simulink model "ee463_project_simulation vol2"  (R2023b)
settings: Solver=VariableStepAuto  StartTime=0.0  StopTime=0.20  RelTol=1e-3
undefined symbols (not defined in the file or in its folder): Acid, Lead
libraries: spsDiodeLib x8, spsACVoltageSourceLib x3, spsSeriesRLCBranchLib x3, spsVoltageMeasurementLib x3, spsBatteryLib x1, spsCurrentMeasurementLib x1, spsGroundLib x1, spsMeanLib x1, spsMosfetLib x1, sps_lib x1
settings Model: Creator=Emir  LastModifiedBy=Emir

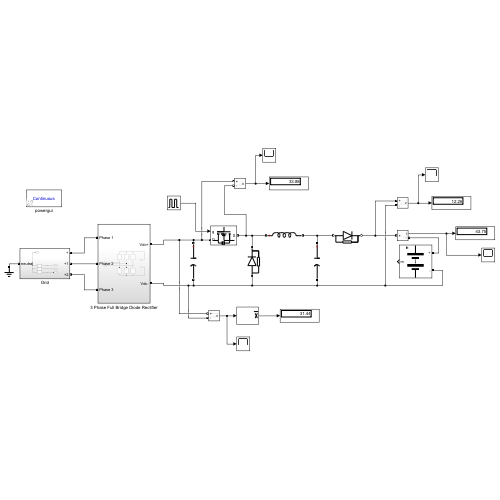
[thumbnail: Simulink's stored preview of the top-level diagram]
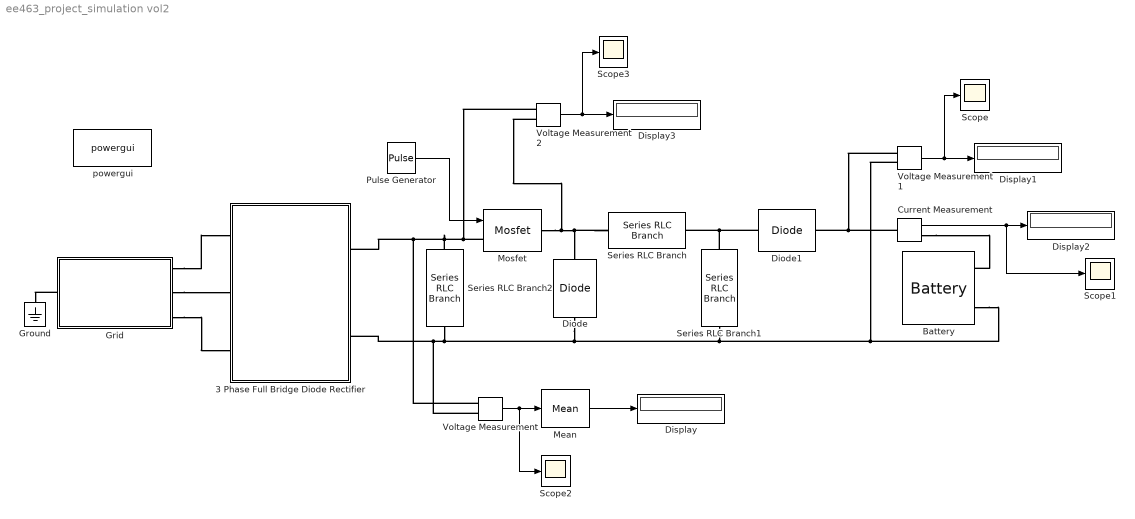
== system ee463_project_simulation vol2 ==
  3 Phase Full Bridge Diode Rectifier : Subsystem
  Battery : spsBatteryLib/Battery  BatType=Lead-Acid  ShowTempParam=off  ThermalPreset=no  ShowAgeParam=off  NomV=12  NomQ=100  SOC=80  Batt_Tr=30  PresetModel=on  MaxQ=104.1667  MinV=9  FullV=13.0658  Dis_rate=20  R=0.0012  Normal_OP=31.0278  expZone="[12.2171     0.333333]"  current=[6.5 13 32.5]  Units=Time  Tci=20  NomT=20  T2=-30  MaxQ2=4.8  FullV2=7.1  Normal_OP2=5.655  expZone2="[6.58           1]"  Rca=0.6  ti=2000  Dp=0  Neq0=0  Tsim=1e6  Ta1=25  Qeol=5.4*0.9  Reol=0.013333*1.2  Char_age=[2.3478, 3]  Dis_age=[2.3478, 10]  N1=1500  N2=10500  N3=1000  N4=1400  Ta2=45  N5=950
  Current Measurement : spsCurrentMeasurementLib/Current Measurement  PhasorSimulation=off  OutputType=Complex  PSBequivalent=0
  Diode : spsDiodeLib/Diode  Ron=0.001  Lon=0  Vf=0.8  IC=0  UseSnubber=0  Rs=500  Cs=250e-9  Measurements=off
  Diode1 : spsDiodeLib/Diode  Ron=0.001  Lon=0  Vf=0.8  IC=0  UseSnubber=0  Rs=500  Cs=250e-9  Measurements=off
  Display{,1..3} (4 alike) : Display
  Grid : Subsystem
  Ground : spsGroundLib/Ground  LConnTagsString=a
  Mean : spsMeanLib/Mean  Freq=60  Vinit=0  Ts=0
  Mosfet : spsMosfetLib/Mosfet  Ron=0.1  Lon=0  Rd=0.01  Vfd=0  IC=0  Rs=1e5  Cs=inf  Measurements=off
  Pulse Generator : DiscretePulseGenerator  PulseType=Time based  Period=1e-5  PulseWidth=50
  Scope{,1..3} (4 alike) : Scope
  Series RLC Branch : spsSeriesRLCBranchLib/Series RLC Branch  LConnTagsString=__new0  RConnTagsString=__new0  BranchType=L  Resistance=1  Inductance=1e-3  SetiL0=off  InitialCurrent=0  Capacitance=1e-6  Setx0=off  InitialVoltage=0  Measurements=None
  Series RLC Branch1 : spsSeriesRLCBranchLib/Series RLC Branch  LConnTagsString=__new0  RConnTagsString=__new0  BranchType=C  Resistance=100  Inductance=1e-3  SetiL0=off  InitialCurrent=0  Capacitance=1000e-6  Setx0=off  InitialVoltage=0  Measurements=None
  Series RLC Branch2 : spsSeriesRLCBranchLib/Series RLC Branch  LConnTagsString=__new0  RConnTagsString=__new0  BranchType=C  Resistance=100  Inductance=1e-3  SetiL0=off  InitialCurrent=0  Capacitance=1000e-6  Setx0=off  InitialVoltage=0  Measurements=None
  Voltage Measurement : spsVoltageMeasurementLib/Voltage Measurement  PhasorSimulation=off  OutputType=Complex  PSBequivalent=0
  Voltage Measurement1 : spsVoltageMeasurementLib/Voltage Measurement  PhasorSimulation=off  OutputType=Complex  PSBequivalent=0
  Voltage Measurement2 : spsVoltageMeasurementLib/Voltage Measurement  PhasorSimulation=off  OutputType=Complex  PSBequivalent=0
  powergui : sps_lib/powergui  Priority=1  SimulationMode=Continuous  SampleTime=50e-6  frequency=60  Iterations=50  frequencyindice=50  Pbase=100e6  ErrMax=1e-4  UnitsV=kV  UnitsW=MW  buscounter=0  FunctionMessages=off  echomessages=off  EnableUseOfTLC=off  CurrentSourceSwitches=off  DisableSnubberDevices=off  DisableRonSwitches=off  DisableVfSwitches=off  DisplayEquations=off  AutomaticDiscreteSolvers=off  SolverType=Tustin/Backward Euler (TBE)  Interpol=off  ExternalGateDelay=off  methode=off  Ts=100  x0status=blocks  SPID=on  SwTol=0  HookPort=off  NonlinearTolerance=1e-4  nMaxIteration=100  ContinueOnMaxIteration=off  RestoreLinks=warning  ResistiveCurrentMeasurement=off  Frange=[0:2:500]  Ylog=off  Xlog=on  ShowGrid=off  save=off  variable=ZData  structure=0  ZoomFFT=off  StartTime=0.0  cycles=1  DisplayStyle=1  fundamental=60  FreqAxis=off  MaxFrequency=1000  frequencyindicesteady=1  RmsSteady=1  display=off
  wires:
  Voltage Measurement/1 -> Scope2/1, Mean/1
  Mean/1 -> Display/1
  Voltage Measurement1/1 -> Scope/1, Display1/1
  Current Measurement/1 -> Scope1/1, Display2/1
  Pulse Generator/1 -> Mosfet/1
  Voltage Measurement2/1 -> Display3/1, Scope3/1
  connections:
  Series RLC Branch2/RConn1 -- Voltage Measurement1/LConn2 -- Battery/LConn2 -- Series RLC Branch1/RConn1 -- Diode/LConn1 -- Voltage Measurement/LConn2 -- 3 Phase Full Bridge Diode Rectifier/RConn2
  Grid/RConn1 -- 3 Phase Full Bridge Diode Rectifier/LConn1
  Grid/RConn2 -- 3 Phase Full Bridge Diode Rectifier/LConn2
  Grid/RConn3 -- 3 Phase Full Bridge Diode Rectifier/LConn3
  Grid/LConn1 -- Ground/LConn1
  Series RLC Branch2/LConn1 -- Voltage Measurement2/LConn1 -- Mosfet/LConn1 -- Voltage Measurement/LConn1 -- 3 Phase Full Bridge Diode Rectifier/RConn1
  Mosfet/RConn1 -- Voltage Measurement2/LConn2 -- Diode/RConn1 -- Series RLC Branch/LConn1
  Series RLC Branch1/LConn1 -- Diode1/LConn1 -- Series RLC Branch/RConn1
  Voltage Measurement1/LConn1 -- Current Measurement/LConn1 -- Diode1/RConn1
  Current Measurement/RConn1 -- Battery/LConn1

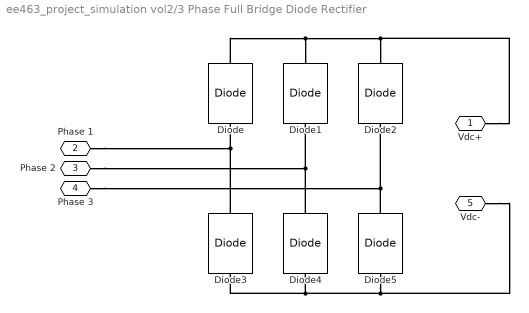
== system ee463_project_simulation vol2/3 Phase Full Bridge Diode Rectifier ==
  Diode{,1..5} (6 alike) : spsDiodeLib/Diode  Ron=0.001  Lon=0  Vf=0.8  IC=0  UseSnubber=0  Rs=500  Cs=250e-9  Measurements=off
  Vdc+ : PMIOPort  Side=Right
  Phase 1 : PMIOPort  Port=2  Side=Left
  Phase 2 : PMIOPort  Port=3  Side=Left
  Phase 3 : PMIOPort  Port=4  Side=Left
  Vdc- : PMIOPort  Port=5  Side=Right
  connections:
  Diode4/RConn1 -- Phase 2/RConn1 -- Diode1/LConn1
  Diode5/RConn1 -- Phase 3/RConn1 -- Diode2/LConn1
  Diode/RConn1 -- Diode1/RConn1 -- Vdc+/RConn1 -- Diode2/RConn1
  Diode3/RConn1 -- Phase 1/RConn1 -- Diode/LConn1
  Diode5/LConn1 -- Vdc-/RConn1 -- Diode4/LConn1 -- Diode3/LConn1

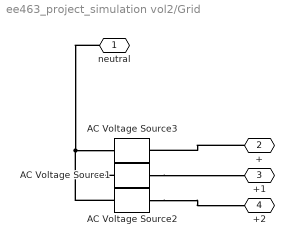
== system ee463_project_simulation vol2/Grid ==
  AC Voltage Source1 : spsACVoltageSourceLib/AC Voltage Source  Amplitude=20  Phase=-120  Frequency=50  SampleTime=0  Measurements=None  BusType=swing  Pref=10e3  Qref=0  Qmin=-inf  Qmax=+inf
  AC Voltage Source2 : spsACVoltageSourceLib/AC Voltage Source  Amplitude=20  Phase=120  Frequency=50  SampleTime=0  Measurements=None  BusType=swing  Pref=10e3  Qref=0  Qmin=-inf  Qmax=+inf
  AC Voltage Source3 : spsACVoltageSourceLib/AC Voltage Source  Amplitude=20  Phase=0  Frequency=50  SampleTime=0  Measurements=None  BusType=swing  Pref=10e3  Qref=0  Qmin=-inf  Qmax=+inf
  neutral : PMIOPort  Side=Left
  + : PMIOPort  Port=2  Side=Right
  +1 : PMIOPort  Port=3  Side=Right
  +2 : PMIOPort  Port=4  Side=Right
  connections:
  AC Voltage Source1/RConn1 -- +1/RConn1
  +/RConn1 -- AC Voltage Source3/RConn1
  AC Voltage Source2/RConn1 -- +2/RConn1
  neutral/RConn1 -- AC Voltage Source2/LConn1 -- AC Voltage Source1/LConn1 -- AC Voltage Source3/LConn1
